simulink library "inp"  (R2021b)
settings: Solver=VariableStepAuto  StartTime=0.0  StopTime=10.0  RelTol=1e-3
undefined symbols (not defined in the file): C_TASK_5MS_S, FALSE, KINP_AcoreReadyToSlp_flg_ovrdflg, KINP_AcoreReadyToSlp_flg_ovrdval, KINP_AllowMovThd_OTA_enum_ovrdflg, KINP_AllowMovThd_OTA_enum_ovrdval, KINP_APSAngleTarget_Deg_ovrdflg, KINP_APSAngleTarget_Deg_ovrdval, KINP_APSDecReq_mps2_ovrdflg, KINP_APSDecReq_mps2_ovrdval, KINP_APSDecReqA_flg_ovrdflg, KINP_APSDecReqA_flg_ovrdval, KINP_APSDFLL_cm_ovrdflg, KINP_APSDFLL_cm_ovrdval, KINP_APSDFLR_cm_ovrdflg, KINP_APSDFLR_cm_ovrdval, KINP_APSDRLL_cm_ovrdflg, KINP_APSDRLL_cm_ovrdval, KINP_APSDRLR_cm_ovrdflg, KINP_APSDRLR_cm_ovrdval, KINP_APSExitCondition_enum_ovrdflg, KINP_APSExitCondition_enum_ovrdval, KINP_APSHWVer_enum_ovrdflg, KINP_APSHWVer_enum_ovrdval, KINP_APSProgressPCT_pct_ovrdflg, KINP_APSProgressPCT_pct_ovrdval, KINP_APSReq_enum_ovrdflg, KINP_APSReq_enum_ovrdval, KINP_APSRQDisplay_enum_ovrdflg, KINP_APSRQDisplay_enum_ovrdval, KINP_APSRqEPASCtrl_flg_ovrdflg, KINP_APSRqEPASCtrl_flg_ovrdval, KINP_APSShiftPosnReq_enum_ovrdval, KINP_APSShiftPosnReq_enum_ovrflg, KINP_APSSpeedCMD_kph_ovrdval, KINP_APSSpeedCMD_kph_ovrflg, KINP_APSStaSystem_enum_ovrdflg, KINP_APSStaSystem_enum_ovrdval, KINP_APSSWVer_enum_ovrdflg, KINP_APSSWVer_enum_ovrdval, KINP_APSVMCReqA_flg_ovrdval, KINP_APSVMCReqA_flg_ovrflg, KINP_APSVRqEPASCtrl_flg_ovrdflg, KINP_APSVRqEPASCtrl_flg_ovrdval, KINP_AuxBattVolmV_mV_ovrdflg, KINP_AuxBattVolmV_mV_ovrdval, KINP_CAASSta_enum_ovrdflg, KINP_CAASSta_enum_ovrdval, KINP_CAASVMCReqA_flg_ovrdval, KINP_CAASVMCReqA_flg_ovrflg, KINP_Chime_enum_ovrdflg, KINP_Chime_enum_ovrdval, KINP_ClearDTCcmd_flg_ovrdflg, KINP_ClearDTCcmd_flg_ovrdval, KINP_EvccAplusPwrUpReq_flg_ovrdflg, KINP_EvccAplusPwrUpReq_flg_ovrdval, KINP_LFID_raw_ovrdval, KINP_LFID_raw_ovrflg, KINP_LRID_raw_ovrdval, KINP_MemOffsetAccX_raw16_ovrdflg ... (+118)
libraries: FVT_lib x503, hcu_lib x1
(part 11 of 16)

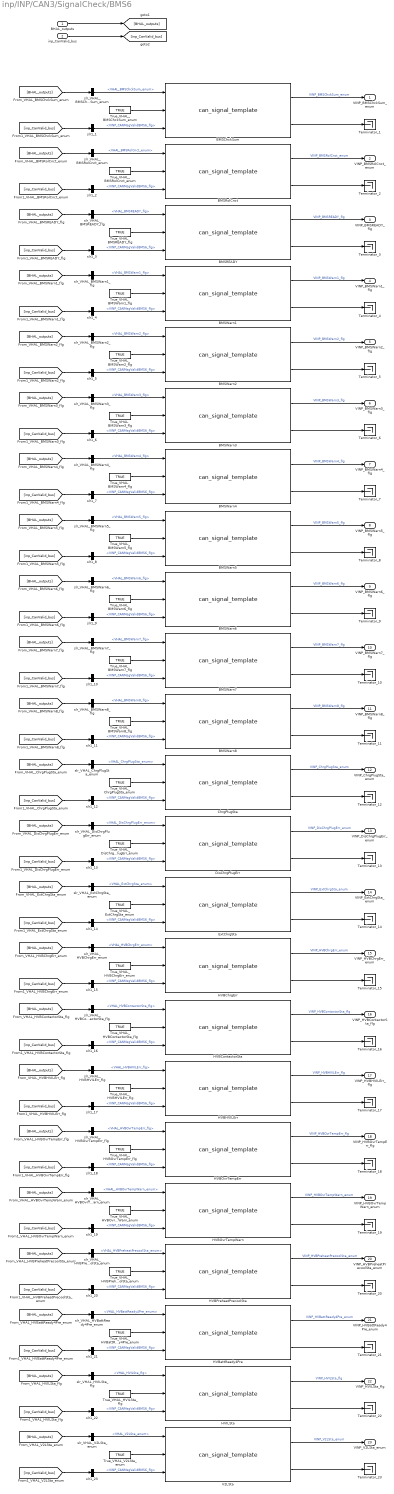
== system inp/INP/CAN3/SignalCheck/BMS6 ==
  BHAL_outputs : Inport
  inp_CanValid_bus : Inport  Port=2
  BMSChckSum : FVT_lib/inp/can_signal_template  SystemSampleTime=-1  VariantActivationTime=update diagram  Latency=0  AutoFrameSizeCalculation=off
      link override defval: Value=KINP_BMSChckSum_enum_defval
      link override ovrdflg: Value=KINP_BMSChckSum_enum_ovrdflg
      link override ovrdval: Value=KINP_BMSChckSum_enum_ovrdval
  BMSREADY : FVT_lib/inp/can_signal_template  SystemSampleTime=-1  VariantActivationTime=update diagram  Latency=0  AutoFrameSizeCalculation=off
      link override defval: Value=KINP_BMSREADY_flg_defval
      link override ovrdflg: Value=KINP_BMSREADY_flg_ovrdflg
      link override ovrdval: Value=KINP_BMSREADY_flg_ovrdval
  BMSRolCnct : FVT_lib/inp/can_signal_template  SystemSampleTime=-1  VariantActivationTime=update diagram  Latency=0  AutoFrameSizeCalculation=off
      link override defval: Value=KINP_BMSRolCnct_enum_defval
      link override ovrdflg: Value=KINP_BMSRolCnct_enum_ovrdflg
      link override ovrdval: Value=KINP_BMSRolCnct_enum_ovrdval
  BMSWarn1 : FVT_lib/inp/can_signal_template  SystemSampleTime=-1  VariantActivationTime=update diagram  Latency=0  AutoFrameSizeCalculation=off
      link override defval: Value=KINP_BMSWarn1_flg_defval
      link override ovrdflg: Value=KINP_BMSWarn1_flg_ovrdflg
      link override ovrdval: Value=KINP_BMSWarn1_flg_ovrdval
  BMSWarn2 : FVT_lib/inp/can_signal_template  SystemSampleTime=-1  VariantActivationTime=update diagram  Latency=0  AutoFrameSizeCalculation=off
      link override defval: Value=KINP_BMSWarn2_flg_defval
      link override ovrdflg: Value=KINP_BMSWarn2_flg_ovrdflg
      link override ovrdval: Value=KINP_BMSWarn2_flg_ovrdval
  BMSWarn3 : FVT_lib/inp/can_signal_template  SystemSampleTime=-1  VariantActivationTime=update diagram  Latency=0  AutoFrameSizeCalculation=off
      link override defval: Value=KINP_BMSWarn3_flg_defval
      link override ovrdflg: Value=KINP_BMSWarn3_flg_ovrdflg
      link override ovrdval: Value=KINP_BMSWarn3_flg_ovrdval
  BMSWarn4 : FVT_lib/inp/can_signal_template  SystemSampleTime=-1  VariantActivationTime=update diagram  Latency=0  AutoFrameSizeCalculation=off
      link override defval: Value=KINP_BMSWarn4_flg_defval
      link override ovrdflg: Value=KINP_BMSWarn4_flg_ovrdflg
      link override ovrdval: Value=KINP_BMSWarn4_flg_ovrdval
  BMSWarn5 : FVT_lib/inp/can_signal_template  SystemSampleTime=-1  VariantActivationTime=update diagram  Latency=0  AutoFrameSizeCalculation=off
      link override defval: Value=KINP_BMSWarn5_flg_defval
      link override ovrdflg: Value=KINP_BMSWarn5_flg_ovrdflg
      link override ovrdval: Value=KINP_BMSWarn5_flg_ovrdval
  BMSWarn6 : FVT_lib/inp/can_signal_template  SystemSampleTime=-1  VariantActivationTime=update diagram  Latency=0  AutoFrameSizeCalculation=off
      link override defval: Value=KINP_BMSWarn6_flg_defval
      link override ovrdflg: Value=KINP_BMSWarn6_flg_ovrdflg
      link override ovrdval: Value=KINP_BMSWarn6_flg_ovrdval
  BMSWarn7 : FVT_lib/inp/can_signal_template  SystemSampleTime=-1  VariantActivationTime=update diagram  Latency=0  AutoFrameSizeCalculation=off
      link override defval: Value=KINP_BMSWarn7_flg_defval
      link override ovrdflg: Value=KINP_BMSWarn7_flg_ovrdflg
      link override ovrdval: Value=KINP_BMSWarn7_flg_ovrdval
  BMSWarn8 : FVT_lib/inp/can_signal_template  SystemSampleTime=-1  VariantActivationTime=update diagram  Latency=0  AutoFrameSizeCalculation=off
      link override defval: Value=KINP_BMSWarn8_flg_defval
      link override ovrdflg: Value=KINP_BMSWarn8_flg_ovrdflg
      link override ovrdval: Value=KINP_BMSWarn8_flg_ovrdval
  ChrgPlugSta : FVT_lib/inp/can_signal_template  SystemSampleTime=-1  VariantActivationTime=update diagram  Latency=0  AutoFrameSizeCalculation=off
      link override defval: Value=KINP_ChrgPlugSta_enum_defval
      link override ovrdflg: Value=KINP_ChrgPlugSta_enum_ovrdflg
      link override ovrdval: Value=KINP_ChrgPlugSta_enum_ovrdval
  DisChrgPlugErr : FVT_lib/inp/can_signal_template  SystemSampleTime=-1  VariantActivationTime=update diagram  Latency=0  AutoFrameSizeCalculation=off
      link override defval: Value=KINP_DisChrgPlugErr_enum_defval
      link override ovrdflg: Value=KINP_DisChrgPlugErr_enum_ovrdflg
      link override ovrdval: Value=KINP_DisChrgPlugErr_enum_ovrdval
  ExtChrgSta : FVT_lib/inp/can_signal_template  SystemSampleTime=-1  VariantActivationTime=update diagram  Latency=0  AutoFrameSizeCalculation=off
      link override defval: Value=KINP_ExtChrgSta_enum_defval
      link override ovrdflg: Value=KINP_ExtChrgSta_enum_ovrdflg
      link override ovrdval: Value=KINP_ExtChrgSta_enum_ovrdval
  HVBChrgErr : FVT_lib/inp/can_signal_template  SystemSampleTime=-1  VariantActivationTime=update diagram  Latency=0  AutoFrameSizeCalculation=off
      link override defval: Value=KINP_HVBChrgErr_enum_defval
      link override ovrdflg: Value=KINP_HVBChrgErr_enum_ovrdflg
      link override ovrdval: Value=KINP_HVBChrgErr_enum_ovrdval
  HVBContactorSta : FVT_lib/inp/can_signal_template  SystemSampleTime=-1  VariantActivationTime=update diagram  Latency=0  AutoFrameSizeCalculation=off
      link override defval: Value=KINP_HVBContactorSta_flg_defval
      link override ovrdflg: Value=KINP_HVBContactorSta_flg_ovrdflg
      link override ovrdval: Value=KINP_HVBContactorSta_flg_ovrdval
  HVBHVILErr : FVT_lib/inp/can_signal_template  SystemSampleTime=-1  VariantActivationTime=update diagram  Latency=0  AutoFrameSizeCalculation=off
      link override defval: Value=KINP_HVBHVILErr_flg_defval
      link override ovrdflg: Value=KINP_HVBHVILErr_flg_ovrdflg
      link override ovrdval: Value=KINP_HVBHVILErr_flg_ovrdval
  HVBOvrTempErr : FVT_lib/inp/can_signal_template  SystemSampleTime=-1  VariantActivationTime=update diagram  Latency=0  AutoFrameSizeCalculation=off
      link override defval: Value=KINP_HVBOvrTempErr_flg_defval
      link override ovrdflg: Value=KINP_HVBOvrTempErr_flg_ovrdflg
      link override ovrdval: Value=KINP_HVBOvrTempErr_flg_ovrdval
  HVBOvrTempWarn : FVT_lib/inp/can_signal_template  SystemSampleTime=-1  VariantActivationTime=update diagram  Latency=0  AutoFrameSizeCalculation=off
      link override defval: Value=KINP_HVBOvrTempWarn_enum_defval
      link override ovrdflg: Value=KINP_HVBOvrTempWarn_enum_ovrdflg
      link override ovrdval: Value=KINP_HVBOvrTempWarn_enum_ovrdval
  HVBPreheatPrecoolSta : FVT_lib/inp/can_signal_template  SystemSampleTime=-1  VariantActivationTime=update diagram  Latency=0  AutoFrameSizeCalculation=off
      link override defval: Value=KINP_HVBPreheatPrecoolSta_enum_defval
      link override ovrdflg: Value=KINP_HVBPreheatPrecoolSta_enum_ovrdflg
      link override ovrdval: Value=KINP_HVBPreheatPrecoolSta_enum_ovrdval
  HVBattReady4Pre : FVT_lib/inp/can_signal_template  SystemSampleTime=-1  VariantActivationTime=update diagram  Latency=0  AutoFrameSizeCalculation=off
      link override defval: Value=KINP_HVBattReady4Pre_enum_defval
      link override ovrdflg: Value=KINP_HVBattReady4Pre_enum_ovrdflg
      link override ovrdval: Value=KINP_HVBattReady4Pre_enum_ovrdval
  HVILSta : FVT_lib/inp/can_signal_template  SystemSampleTime=-1  VariantActivationTime=update diagram  Latency=0  AutoFrameSizeCalculation=off
      link override defval: Value=KINP_HVILSta_flg_defval
      link override ovrdflg: Value=KINP_HVILSta_flg_ovrdflg
      link override ovrdval: Value=KINP_HVILSta_flg_ovrdval
  Terminator_{1..23} (23 alike) : Terminator
  True_VHAL_BMSChckSum_enum : Constant  Value=TRUE  OutDataTypeStr=boolean
  True_VHAL_BMSREADY_flg : Constant  Value=TRUE  OutDataTypeStr=boolean
  True_VHAL_BMSRolCnct_enum : Constant  Value=TRUE  OutDataTypeStr=boolean
  True_VHAL_BMSWarn1_flg : Constant  Value=TRUE  OutDataTypeStr=boolean
  True_VHAL_BMSWarn2_flg : Constant  Value=TRUE  OutDataTypeStr=boolean
  True_VHAL_BMSWarn3_flg : Constant  Value=TRUE  OutDataTypeStr=boolean
  True_VHAL_BMSWarn4_flg : Constant  Value=TRUE  OutDataTypeStr=boolean
  True_VHAL_BMSWarn5_flg : Constant  Value=TRUE  OutDataTypeStr=boolean
  True_VHAL_BMSWarn6_flg : Constant  Value=TRUE  OutDataTypeStr=boolean
  True_VHAL_BMSWarn7_flg : Constant  Value=TRUE  OutDataTypeStr=boolean
  True_VHAL_BMSWarn8_flg : Constant  Value=TRUE  OutDataTypeStr=boolean
  True_VHAL_ChrgPlugSta_enum : Constant  Value=TRUE  OutDataTypeStr=boolean
  True_VHAL_DisChrgPlugErr_enum : Constant  Value=TRUE  OutDataTypeStr=boolean
  True_VHAL_ExtChrgSta_enum : Constant  Value=TRUE  OutDataTypeStr=boolean
  True_VHAL_HVBChrgErr_enum : Constant  Value=TRUE  OutDataTypeStr=boolean
  True_VHAL_HVBContactorSta_flg : Constant  Value=TRUE  OutDataTypeStr=boolean
  True_VHAL_HVBHVILErr_flg : Constant  Value=TRUE  OutDataTypeStr=boolean
  True_VHAL_HVBOvrTempErr_flg : Constant  Value=TRUE  OutDataTypeStr=boolean
  True_VHAL_HVBOvrTempWarn_enum : Constant  Value=TRUE  OutDataTypeStr=boolean
  True_VHAL_HVBPreheatPrecoolSta_enum : Constant  Value=TRUE  OutDataTypeStr=boolean
  True_VHAL_HVBattReady4Pre_enum : Constant  Value=TRUE  OutDataTypeStr=boolean
  True_VHAL_HVILSta_flg : Constant  Value=TRUE  OutDataTypeStr=boolean
  True_VHAL_V2LSta_enum : Constant  Value=TRUE  OutDataTypeStr=boolean
  V2LSta : FVT_lib/inp/can_signal_template  SystemSampleTime=-1  VariantActivationTime=update diagram  Latency=0  AutoFrameSizeCalculation=off
      link override defval: Value=KINP_V2LSta_enum_defval
      link override ovrdflg: Value=KINP_V2LSta_enum_ovrdflg
      link override ovrdval: Value=KINP_V2LSta_enum_ovrdval
  slr1_{1..23} (23 alike) : BusSelector  OutputSignals=VINP_CANMsgValidBMS6_flg
  slr_VHAL_BMSChckSum_enum : BusSelector  OutputSignals=VHAL_BMSChckSum_enum
  slr_VHAL_BMSREADY_flg : BusSelector  OutputSignals=VHAL_BMSREADY_flg
  slr_VHAL_BMSRolCnct_enum : BusSelector  OutputSignals=VHAL_BMSRolCnct_enum
  slr_VHAL_BMSWarn1_flg : BusSelector  OutputSignals=VHAL_BMSWarn1_flg
  slr_VHAL_BMSWarn2_flg : BusSelector  OutputSignals=VHAL_BMSWarn2_flg
  slr_VHAL_BMSWarn3_flg : BusSelector  OutputSignals=VHAL_BMSWarn3_flg
  slr_VHAL_BMSWarn4_flg : BusSelector  OutputSignals=VHAL_BMSWarn4_flg
  slr_VHAL_BMSWarn5_flg : BusSelector  OutputSignals=VHAL_BMSWarn5_flg
  slr_VHAL_BMSWarn6_flg : BusSelector  OutputSignals=VHAL_BMSWarn6_flg
  slr_VHAL_BMSWarn7_flg : BusSelector  OutputSignals=VHAL_BMSWarn7_flg
  slr_VHAL_BMSWarn8_flg : BusSelector  OutputSignals=VHAL_BMSWarn8_flg
  slr_VHAL_ChrgPlugSta_enum : BusSelector  OutputSignals=VHAL_ChrgPlugSta_enum
  slr_VHAL_DisChrgPlugErr_enum : BusSelector  OutputSignals=VHAL_DisChrgPlugErr_enum
  slr_VHAL_ExtChrgSta_enum : BusSelector  OutputSignals=VHAL_ExtChrgSta_enum
  slr_VHAL_HVBChrgErr_enum : BusSelector  OutputSignals=VHAL_HVBChrgErr_enum
  slr_VHAL_HVBContactorSta_flg : BusSelector  OutputSignals=VHAL_HVBContactorSta_flg
  slr_VHAL_HVBHVILErr_flg : BusSelector  OutputSignals=VHAL_HVBHVILErr_flg
  slr_VHAL_HVBOvrTempErr_flg : BusSelector  OutputSignals=VHAL_HVBOvrTempErr_flg
  slr_VHAL_HVBOvrTempWarn_enum : BusSelector  OutputSignals=VHAL_HVBOvrTempWarn_enum
  slr_VHAL_HVBPreheatPrecoolSta_enum : BusSelector  OutputSignals=VHAL_HVBPreheatPrecoolSta_enum
  slr_VHAL_HVBattReady4Pre_enum : BusSelector  OutputSignals=VHAL_HVBattReady4Pre_enum
  slr_VHAL_HVILSta_flg : BusSelector  OutputSignals=VHAL_HVILSta_flg
  slr_VHAL_V2LSta_enum : BusSelector  OutputSignals=VHAL_V2LSta_enum
  VINP_BMSChckSum_enum : Outport
  VINP_BMSRolCnct_enum : Outport  Port=2
  VINP_BMSREADY_flg : Outport  Port=3
  VINP_BMSWarn1_flg : Outport  Port=4
  VINP_BMSWarn2_flg : Outport  Port=5
  VINP_BMSWarn3_flg : Outport  Port=6
  VINP_BMSWarn4_flg : Outport  Port=7
  VINP_BMSWarn5_flg : Outport  Port=8
  VINP_BMSWarn6_flg : Outport  Port=9
  VINP_BMSWarn7_flg : Outport  Port=10
  VINP_BMSWarn8_flg : Outport  Port=11
  VINP_ChrgPlugSta_enum : Outport  Port=12
  VINP_DisChrgPlugErr_enum : Outport  Port=13
  VINP_ExtChrgSta_enum : Outport  Port=14
  VINP_HVBChrgErr_enum : Outport  Port=15
  VINP_HVBContactorSta_flg : Outport  Port=16
  VINP_HVBHVILErr_flg : Outport  Port=17
  VINP_HVBOvrTempErr_flg : Outport  Port=18
  VINP_HVBOvrTempWarn_enum : Outport  Port=19
  VINP_HVBPreheatPrecoolSta_enum : Outport  Port=20
  VINP_HVBattReady4Pre_enum : Outport  Port=21
  VINP_HVILSta_flg : Outport  Port=22
  VINP_V2LSta_enum : Outport  Port=23
  wires:
  BHAL_outputs/1 -> [BHAL_outputs]
  inp_CanValid_bus/1 -> [inp_CanValid_bus]
  [BHAL_outputs] -> slr_VHAL_BMSChckSum_enum/1
  slr_VHAL_BMSChckSum_enum/1 -> BMSChckSum/1  "<VHAL_BMSChckSum_enum>"
  True_VHAL_BMSChckSum_enum/1 -> BMSChckSum/2
  [inp_CanValid_bus] -> slr1_1/1
  slr1_1/1 -> BMSChckSum/3  "<VINP_CANMsgValidBMS6_flg>"
  BMSChckSum/1 -> VINP_BMSChckSum_enum/1  "VINP_BMSChckSum_enum"
  BMSChckSum/2 -> Terminator_1/1
  [BHAL_outputs] -> slr_VHAL_BMSRolCnct_enum/1
  slr_VHAL_BMSRolCnct_enum/1 -> BMSRolCnct/1  "<VHAL_BMSRolCnct_enum>"
  True_VHAL_BMSRolCnct_enum/1 -> BMSRolCnct/2
  [inp_CanValid_bus] -> slr1_2/1
  slr1_2/1 -> BMSRolCnct/3  "<VINP_CANMsgValidBMS6_flg>"
  BMSRolCnct/1 -> VINP_BMSRolCnct_enum/1  "VINP_BMSRolCnct_enum"
  BMSRolCnct/2 -> Terminator_2/1
  [BHAL_outputs] -> slr_VHAL_BMSREADY_flg/1
  slr_VHAL_BMSREADY_flg/1 -> BMSREADY/1  "<VHAL_BMSREADY_flg>"
  True_VHAL_BMSREADY_flg/1 -> BMSREADY/2
  [inp_CanValid_bus] -> slr1_3/1
  slr1_3/1 -> BMSREADY/3  "<VINP_CANMsgValidBMS6_flg>"
  BMSREADY/1 -> VINP_BMSREADY_flg/1  "VINP_BMSREADY_flg"
  BMSREADY/2 -> Terminator_3/1
  [BHAL_outputs] -> slr_VHAL_BMSWarn1_flg/1
  slr_VHAL_BMSWarn1_flg/1 -> BMSWarn1/1  "<VHAL_BMSWarn1_flg>"
  True_VHAL_BMSWarn1_flg/1 -> BMSWarn1/2
  [inp_CanValid_bus] -> slr1_4/1
  slr1_4/1 -> BMSWarn1/3  "<VINP_CANMsgValidBMS6_flg>"
  BMSWarn1/1 -> VINP_BMSWarn1_flg/1  "VINP_BMSWarn1_flg"
  BMSWarn1/2 -> Terminator_4/1
  [BHAL_outputs] -> slr_VHAL_BMSWarn2_flg/1
  slr_VHAL_BMSWarn2_flg/1 -> BMSWarn2/1  "<VHAL_BMSWarn2_flg>"
  True_VHAL_BMSWarn2_flg/1 -> BMSWarn2/2
  [inp_CanValid_bus] -> slr1_5/1
  slr1_5/1 -> BMSWarn2/3  "<VINP_CANMsgValidBMS6_flg>"
  BMSWarn2/1 -> VINP_BMSWarn2_flg/1  "VINP_BMSWarn2_flg"
  BMSWarn2/2 -> Terminator_5/1
  [BHAL_outputs] -> slr_VHAL_BMSWarn3_flg/1
  slr_VHAL_BMSWarn3_flg/1 -> BMSWarn3/1  "<VHAL_BMSWarn3_flg>"
  True_VHAL_BMSWarn3_flg/1 -> BMSWarn3/2
  [inp_CanValid_bus] -> slr1_6/1
  slr1_6/1 -> BMSWarn3/3  "<VINP_CANMsgValidBMS6_flg>"
  BMSWarn3/1 -> VINP_BMSWarn3_flg/1  "VINP_BMSWarn3_flg"
  BMSWarn3/2 -> Terminator_6/1
  [BHAL_outputs] -> slr_VHAL_BMSWarn4_flg/1
  slr_VHAL_BMSWarn4_flg/1 -> BMSWarn4/1  "<VHAL_BMSWarn4_flg>"
  True_VHAL_BMSWarn4_flg/1 -> BMSWarn4/2
  [inp_CanValid_bus] -> slr1_7/1
  slr1_7/1 -> BMSWarn4/3  "<VINP_CANMsgValidBMS6_flg>"
  BMSWarn4/1 -> VINP_BMSWarn4_flg/1  "VINP_BMSWarn4_flg"
  BMSWarn4/2 -> Terminator_7/1
  [BHAL_outputs] -> slr_VHAL_BMSWarn5_flg/1
  slr_VHAL_BMSWarn5_flg/1 -> BMSWarn5/1  "<VHAL_BMSWarn5_flg>"
  True_VHAL_BMSWarn5_flg/1 -> BMSWarn5/2
  [inp_CanValid_bus] -> slr1_8/1
  slr1_8/1 -> BMSWarn5/3  "<VINP_CANMsgValidBMS6_flg>"
  BMSWarn5/1 -> VINP_BMSWarn5_flg/1  "VINP_BMSWarn5_flg"
  BMSWarn5/2 -> Terminator_8/1
  [BHAL_outputs] -> slr_VHAL_BMSWarn6_flg/1
  slr_VHAL_BMSWarn6_flg/1 -> BMSWarn6/1  "<VHAL_BMSWarn6_flg>"
  True_VHAL_BMSWarn6_flg/1 -> BMSWarn6/2
  [inp_CanValid_bus] -> slr1_9/1
  slr1_9/1 -> BMSWarn6/3  "<VINP_CANMsgValidBMS6_flg>"
  BMSWarn6/1 -> VINP_BMSWarn6_flg/1  "VINP_BMSWarn6_flg"
  BMSWarn6/2 -> Terminator_9/1
  [BHAL_outputs] -> slr_VHAL_BMSWarn7_flg/1
  slr_VHAL_BMSWarn7_flg/1 -> BMSWarn7/1  "<VHAL_BMSWarn7_flg>"
  True_VHAL_BMSWarn7_flg/1 -> BMSWarn7/2
  [inp_CanValid_bus] -> slr1_10/1
  slr1_10/1 -> BMSWarn7/3  "<VINP_CANMsgValidBMS6_flg>"
  BMSWarn7/1 -> VINP_BMSWarn7_flg/1  "VINP_BMSWarn7_flg"
  BMSWarn7/2 -> Terminator_10/1
  [BHAL_outputs] -> slr_VHAL_BMSWarn8_flg/1
  slr_VHAL_BMSWarn8_flg/1 -> BMSWarn8/1  "<VHAL_BMSWarn8_flg>"
  True_VHAL_BMSWarn8_flg/1 -> BMSWarn8/2
  [inp_CanValid_bus] -> slr1_11/1
  slr1_11/1 -> BMSWarn8/3  "<VINP_CANMsgValidBMS6_flg>"
  BMSWarn8/1 -> VINP_BMSWarn8_flg/1  "VINP_BMSWarn8_flg"
  BMSWarn8/2 -> Terminator_11/1
  [BHAL_outputs] -> slr_VHAL_ChrgPlugSta_enum/1
  slr_VHAL_ChrgPlugSta_enum/1 -> ChrgPlugSta/1  "<VHAL_ChrgPlugSta_enum>"
  True_VHAL_ChrgPlugSta_enum/1 -> ChrgPlugSta/2
  [inp_CanValid_bus] -> slr1_12/1
  slr1_12/1 -> ChrgPlugSta/3  "<VINP_CANMsgValidBMS6_flg>"
  ChrgPlugSta/1 -> VINP_ChrgPlugSta_enum/1  "VINP_ChrgPlugSta_enum"
  ChrgPlugSta/2 -> Terminator_12/1
  [BHAL_outputs] -> slr_VHAL_DisChrgPlugErr_enum/1
  slr_VHAL_DisChrgPlugErr_enum/1 -> DisChrgPlugErr/1  "<VHAL_DisChrgPlugErr_enum>"
  True_VHAL_DisChrgPlugErr_enum/1 -> DisChrgPlugErr/2
  [inp_CanValid_bus] -> slr1_13/1
  slr1_13/1 -> DisChrgPlugErr/3  "<VINP_CANMsgValidBMS6_flg>"
  DisChrgPlugErr/1 -> VINP_DisChrgPlugErr_enum/1  "VINP_DisChrgPlugErr_enum"
  DisChrgPlugErr/2 -> Terminator_13/1
  [BHAL_outputs] -> slr_VHAL_ExtChrgSta_enum/1
  slr_VHAL_ExtChrgSta_enum/1 -> ExtChrgSta/1  "<VHAL_ExtChrgSta_enum>"
  True_VHAL_ExtChrgSta_enum/1 -> ExtChrgSta/2
  [inp_CanValid_bus] -> slr1_14/1
  slr1_14/1 -> ExtChrgSta/3  "<VINP_CANMsgValidBMS6_flg>"
  ExtChrgSta/1 -> VINP_ExtChrgSta_enum/1  "VINP_ExtChrgSta_enum"
  ExtChrgSta/2 -> Terminator_14/1
  [BHAL_outputs] -> slr_VHAL_HVBChrgErr_enum/1
  slr_VHAL_HVBChrgErr_enum/1 -> HVBChrgErr/1  "<VHAL_HVBChrgErr_enum>"
  True_VHAL_HVBChrgErr_enum/1 -> HVBChrgErr/2
  [inp_CanValid_bus] -> slr1_15/1
  slr1_15/1 -> HVBChrgErr/3  "<VINP_CANMsgValidBMS6_flg>"
  HVBChrgErr/1 -> VINP_HVBChrgErr_enum/1  "VINP_HVBChrgErr_enum"
  HVBChrgErr/2 -> Terminator_15/1
  [BHAL_outputs] -> slr_VHAL_HVBContactorSta_flg/1
  slr_VHAL_HVBContactorSta_flg/1 -> HVBContactorSta/1  "<VHAL_HVBContactorSta_flg>"
  True_VHAL_HVBContactorSta_flg/1 -> HVBContactorSta/2
  [inp_CanValid_bus] -> slr1_16/1
  slr1_16/1 -> HVBContactorSta/3  "<VINP_CANMsgValidBMS6_flg>"
  HVBContactorSta/1 -> VINP_HVBContactorSta_flg/1  "VINP_HVBContactorSta_flg"
  HVBContactorSta/2 -> Terminator_16/1
  [BHAL_outputs] -> slr_VHAL_HVBHVILErr_flg/1
  slr_VHAL_HVBHVILErr_flg/1 -> HVBHVILErr/1  "<VHAL_HVBHVILErr_flg>"
  True_VHAL_HVBHVILErr_flg/1 -> HVBHVILErr/2
  [inp_CanValid_bus] -> slr1_17/1
  slr1_17/1 -> HVBHVILErr/3  "<VINP_CANMsgValidBMS6_flg>"
  HVBHVILErr/1 -> VINP_HVBHVILErr_flg/1  "VINP_HVBHVILErr_flg"
  HVBHVILErr/2 -> Terminator_17/1
  [BHAL_outputs] -> slr_VHAL_HVBOvrTempErr_flg/1
  slr_VHAL_HVBOvrTempErr_flg/1 -> HVBOvrTempErr/1  "<VHAL_HVBOvrTempErr_flg>"
  True_VHAL_HVBOvrTempErr_flg/1 -> HVBOvrTempErr/2
  [inp_CanValid_bus] -> slr1_18/1
  slr1_18/1 -> HVBOvrTempErr/3  "<VINP_CANMsgValidBMS6_flg>"
  HVBOvrTempErr/1 -> VINP_HVBOvrTempErr_flg/1  "VINP_HVBOvrTempErr_flg"
  HVBOvrTempErr/2 -> Terminator_18/1
  [BHAL_outputs] -> slr_VHAL_HVBOvrTempWarn_enum/1
  slr_VHAL_HVBOvrTempWarn_enum/1 -> HVBOvrTempWarn/1  "<VHAL_HVBOvrTempWarn_enum>"
  True_VHAL_HVBOvrTempWarn_enum/1 -> HVBOvrTempWarn/2
  [inp_CanValid_bus] -> slr1_19/1
  slr1_19/1 -> HVBOvrTempWarn/3  "<VINP_CANMsgValidBMS6_flg>"
  HVBOvrTempWarn/1 -> VINP_HVBOvrTempWarn_enum/1  "VINP_HVBOvrTempWarn_enum"
  HVBOvrTempWarn/2 -> Terminator_19/1
  [BHAL_outputs] -> slr_VHAL_HVBPreheatPrecoolSta_enum/1
  slr_VHAL_HVBPreheatPrecoolSta_enum/1 -> HVBPreheatPrecoolSta/1  "<VHAL_HVBPreheatPrecoolSta_enum>"
  True_VHAL_HVBPreheatPrecoolSta_enum/1 -> HVBPreheatPrecoolSta/2
  [inp_CanValid_bus] -> slr1_20/1
  slr1_20/1 -> HVBPreheatPrecoolSta/3  "<VINP_CANMsgValidBMS6_flg>"
  HVBPreheatPrecoolSta/1 -> VINP_HVBPreheatPrecoolSta_enum/1  "VINP_HVBPreheatPrecoolSta_enum"
  HVBPreheatPrecoolSta/2 -> Terminator_20/1
  [BHAL_outputs] -> slr_VHAL_HVBattReady4Pre_enum/1
  slr_VHAL_HVBattReady4Pre_enum/1 -> HVBattReady4Pre/1  "<VHAL_HVBattReady4Pre_enum>"
  True_VHAL_HVBattReady4Pre_enum/1 -> HVBattReady4Pre/2
  [inp_CanValid_bus] -> slr1_21/1
  slr1_21/1 -> HVBattReady4Pre/3  "<VINP_CANMsgValidBMS6_flg>"
  HVBattReady4Pre/1 -> VINP_HVBattReady4Pre_enum/1  "VINP_HVBattReady4Pre_enum"
  HVBattReady4Pre/2 -> Terminator_21/1
  [BHAL_outputs] -> slr_VHAL_HVILSta_flg/1
  slr_VHAL_HVILSta_flg/1 -> HVILSta/1  "<VHAL_HVILSta_flg>"
  True_VHAL_HVILSta_flg/1 -> HVILSta/2
  [inp_CanValid_bus] -> slr1_22/1
  slr1_22/1 -> HVILSta/3  "<VINP_CANMsgValidBMS6_flg>"
  HVILSta/1 -> VINP_HVILSta_flg/1  "VINP_HVILSta_flg"
  HVILSta/2 -> Terminator_22/1
  [BHAL_outputs] -> slr_VHAL_V2LSta_enum/1
  slr_VHAL_V2LSta_enum/1 -> V2LSta/1  "<VHAL_V2LSta_enum>"
  True_VHAL_V2LSta_enum/1 -> V2LSta/2
  [inp_CanValid_bus] -> slr1_23/1
  slr1_23/1 -> V2LSta/3  "<VINP_CANMsgValidBMS6_flg>"
  V2LSta/1 -> VINP_V2LSta_enum/1  "VINP_V2LSta_enum"
  V2LSta/2 -> Terminator_23/1

== system inp/INP/CAN3/SignalCheck/BMS8 ==
  BHAL_outputs : Inport
  inp_CanValid_bus : Inport  Port=2
  MainRlyNegSta : FVT_lib/inp/can_signal_template  SystemSampleTime=-1  VariantActivationTime=update diagram  Latency=0  AutoFrameSizeCalculation=off
      link override defval: Value=KINP_MainRlyNegSta_enum_defval
      link override ovrdflg: Value=KINP_MainRlyNegSta_enum_ovrdflg
      link override ovrdval: Value=KINP_MainRlyNegSta_enum_ovrdval
  MainRlyPosSta : FVT_lib/inp/can_signal_template  SystemSampleTime=-1  VariantActivationTime=update diagram  Latency=0  AutoFrameSizeCalculation=off
      link override defval: Value=KINP_MainRlyPosSta_enum_defval
      link override ovrdflg: Value=KINP_MainRlyPosSta_enum_ovrdflg
      link override ovrdval: Value=KINP_MainRlyPosSta_enum_ovrdval
  Terminator_1 : Terminator
  Terminator_2 : Terminator
  True_VHAL_MainRlyNegSta_enum : Constant  Value=TRUE  OutDataTypeStr=boolean
  True_VHAL_MainRlyPosSta_enum : Constant  Value=TRUE  OutDataTypeStr=boolean
  slr1_1 : BusSelector  OutputSignals=VINP_CANMsgValidBMS8_flg
  slr1_2 : BusSelector  OutputSignals=VINP_CANMsgValidBMS8_flg
  slr_VHAL_MainRlyNegSta_enum : BusSelector  OutputSignals=VHAL_MainRlyNegSta_enum
  slr_VHAL_MainRlyPosSta_enum : BusSelector  OutputSignals=VHAL_MainRlyPosSta_enum
  VINP_MainRlyNegSta_enum : Outport
  VINP_MainRlyPosSta_enum : Outport  Port=2
  wires:
  BHAL_outputs/1 -> [BHAL_outputs]
  inp_CanValid_bus/1 -> [inp_CanValid_bus]
  [BHAL_outputs] -> slr_VHAL_MainRlyNegSta_enum/1
  slr_VHAL_MainRlyNegSta_enum/1 -> MainRlyNegSta/1  "<VHAL_MainRlyNegSta_enum>"
  True_VHAL_MainRlyNegSta_enum/1 -> MainRlyNegSta/2
  [inp_CanValid_bus] -> slr1_1/1
  slr1_1/1 -> MainRlyNegSta/3  "<VINP_CANMsgValidBMS8_flg>"
  MainRlyNegSta/1 -> VINP_MainRlyNegSta_enum/1  "VINP_MainRlyNegSta_enum"
  MainRlyNegSta/2 -> Terminator_1/1
  [BHAL_outputs] -> slr_VHAL_MainRlyPosSta_enum/1
  slr_VHAL_MainRlyPosSta_enum/1 -> MainRlyPosSta/1  "<VHAL_MainRlyPosSta_enum>"
  True_VHAL_MainRlyPosSta_enum/1 -> MainRlyPosSta/2
  [inp_CanValid_bus] -> slr1_2/1
  slr1_2/1 -> MainRlyPosSta/3  "<VINP_CANMsgValidBMS8_flg>"
  MainRlyPosSta/1 -> VINP_MainRlyPosSta_enum/1  "VINP_MainRlyPosSta_enum"
  MainRlyPosSta/2 -> Terminator_2/1

== system inp/INP/CAN3/SignalCheck/CCU1 ==
  BHAL_outputs : Inport
  inp_CanValid_bus : Inport  Port=2
  CSCCU1 : FVT_lib/inp/can_signal_template  SystemSampleTime=-1  VariantActivationTime=update diagram  Latency=0  AutoFrameSizeCalculation=off
      link override defval: Value=KINP_CSCCU1_enum_defval
      link override ovrdflg: Value=KINP_CSCCU1_enum_ovrdflg
      link override ovrdval: Value=KINP_CSCCU1_enum_ovrdval
  DCDCAuxCur : FVT_lib/inp/can_signal_template  SystemSampleTime=-1  VariantActivationTime=update diagram  Latency=0  AutoFrameSizeCalculation=off
      link override defval: Value=KINP_DCDCAuxCur_A_defval
      link override ovrdflg: Value=KINP_DCDCAuxCur_A_ovrdflg
      link override ovrdval: Value=KINP_DCDCAuxCur_A_ovrdval
  DCDCAuxVolt : FVT_lib/inp/can_signal_template  SystemSampleTime=-1  VariantActivationTime=update diagram  Latency=0  AutoFrameSizeCalculation=off
      link override defval: Value=KINP_DCDCAuxVolt_V_defval
      link override ovrdflg: Value=KINP_DCDCAuxVolt_V_ovrdflg
      link override ovrdval: Value=KINP_DCDCAuxVolt_V_ovrdval
  DCDCHVCur : FVT_lib/inp/can_signal_template  SystemSampleTime=-1  VariantActivationTime=update diagram  Latency=0  AutoFrameSizeCalculation=off
      link override defval: Value=KINP_DCDCHVCur_A_defval
      link override ovrdflg: Value=KINP_DCDCHVCur_A_ovrdflg
      link override ovrdval: Value=KINP_DCDCHVCur_A_ovrdval
  DCDCInVoltInf : FVT_lib/inp/can_signal_template  SystemSampleTime=-1  VariantActivationTime=update diagram  Latency=0  AutoFrameSizeCalculation=off
      link override defval: Value=KINP_DCDCInVoltInf_V_defval
      link override ovrdflg: Value=KINP_DCDCInVoltInf_V_ovrdflg
      link override ovrdval: Value=KINP_DCDCInVoltInf_V_ovrdval
  DCDCPreCompleted : FVT_lib/inp/can_signal_template  SystemSampleTime=-1  VariantActivationTime=update diagram  Latency=0  AutoFrameSizeCalculation=off
      link override defval: Value=KINP_DCDCPreCompleted_enum_defval
      link override ovrdflg: Value=KINP_DCDCPreCompleted_enum_ovrdflg
      link override ovrdval: Value=KINP_DCDCPreCompleted_enum_ovrdval
  OBCDCCurrInf : FVT_lib/inp/can_signal_template  SystemSampleTime=-1  VariantActivationTime=update diagram  Latency=0  AutoFrameSizeCalculation=off
      link override defval: Value=KINP_OBCDCCurrInf_A_defval
      link override ovrdflg: Value=KINP_OBCDCCurrInf_A_ovrdflg
      link override ovrdval: Value=KINP_OBCDCCurrInf_A_ovrdval
  OBCDCVoltInf : FVT_lib/inp/can_signal_template  SystemSampleTime=-1  VariantActivationTime=update diagram  Latency=0  AutoFrameSizeCalculation=off
      link override defval: Value=KINP_OBCDCVoltInf_V_defval
      link override ovrdflg: Value=KINP_OBCDCVoltInf_V_ovrdflg
      link override ovrdval: Value=KINP_OBCDCVoltInf_V_ovrdval
  OBCPreCompleted : FVT_lib/inp/can_signal_template  SystemSampleTime=-1  VariantActivationTime=update diagram  Latency=0  AutoFrameSizeCalculation=off
      link override defval: Value=KINP_OBCPreCompleted_enum_defval
      link override ovrdflg: Value=KINP_OBCPreCompleted_enum_ovrdflg
      link override ovrdval: Value=KINP_OBCPreCompleted_enum_ovrdval
  OBCWakeup4Plugin : FVT_lib/inp/can_signal_template  SystemSampleTime=-1  VariantActivationTime=update diagram  Latency=0  AutoFrameSizeCalculation=off
      link override defval: Value=KINP_OBCWakeup4Plugin_flg_defval
      link override ovrdflg: Value=KINP_OBCWakeup4Plugin_flg_ovrdflg
      link override ovrdval: Value=KINP_OBCWakeup4Plugin_flg_ovrdval
  RCCCU1 : FVT_lib/inp/can_signal_template  SystemSampleTime=-1  VariantActivationTime=update diagram  Latency=0  AutoFrameSizeCalculation=off
      link override defval: Value=KINP_RCCCU1_enum_defval
      link override ovrdflg: Value=KINP_RCCCU1_enum_ovrdflg
      link override ovrdval: Value=KINP_RCCCU1_enum_ovrdval
  Terminator_{1..11} (11 alike) : Terminator
  True_VHAL_CSCCU1_enum : Constant  Value=TRUE  OutDataTypeStr=boolean
  True_VHAL_DCDCAuxCur_A : Constant  Value=TRUE  OutDataTypeStr=boolean
  True_VHAL_DCDCAuxVolt_V : Constant  Value=TRUE  OutDataTypeStr=boolean
  True_VHAL_DCDCHVCur_A : Constant  Value=TRUE  OutDataTypeStr=boolean
  True_VHAL_DCDCInVoltInf_V : Constant  Value=TRUE  OutDataTypeStr=boolean
  True_VHAL_DCDCPreCompleted_enum : Constant  Value=TRUE  OutDataTypeStr=boolean
  True_VHAL_OBCDCCurrInf_A : Constant  Value=TRUE  OutDataTypeStr=boolean
  True_VHAL_OBCDCVoltInf_V : Constant  Value=TRUE  OutDataTypeStr=boolean
  True_VHAL_OBCPreCompleted_enum : Constant  Value=TRUE  OutDataTypeStr=boolean
  True_VHAL_OBCWakeup4Plugin_flg : Constant  Value=TRUE  OutDataTypeStr=boolean
  True_VHAL_RCCCU1_enum : Constant  Value=TRUE  OutDataTypeStr=boolean
  slr1_{1..11} (11 alike) : BusSelector  OutputSignals=VINP_CANMsgValidCCU1_flg
  slr_VHAL_CSCCU1_enum : BusSelector  OutputSignals=VHAL_CSCCU1_enum
  slr_VHAL_DCDCAuxCur_A : BusSelector  OutputSignals=VHAL_DCDCAuxCur_A
  slr_VHAL_DCDCAuxVolt_V : BusSelector  OutputSignals=VHAL_DCDCAuxVolt_V
  slr_VHAL_DCDCHVCur_A : BusSelector  OutputSignals=VHAL_DCDCHVCur_A
  slr_VHAL_DCDCInVoltInf_V : BusSelector  OutputSignals=VHAL_DCDCInVoltInf_V
  slr_VHAL_DCDCPreCompleted_enum : BusSelector  OutputSignals=VHAL_DCDCPreCompleted_enum
  slr_VHAL_OBCDCCurrInf_A : BusSelector  OutputSignals=VHAL_OBCDCCurrInf_A
  slr_VHAL_OBCDCVoltInf_V : BusSelector  OutputSignals=VHAL_OBCDCVoltInf_V
  slr_VHAL_OBCPreCompleted_enum : BusSelector  OutputSignals=VHAL_OBCPreCompleted_enum
  slr_VHAL_OBCWakeup4Plugin_flg : BusSelector  OutputSignals=VHAL_OBCWakeup4Plugin_flg
  slr_VHAL_RCCCU1_enum : BusSelector  OutputSignals=VHAL_RCCCU1_enum
  VINP_CSCCU1_enum : Outport
  VINP_DCDCAuxCur_A : Outport  Port=2
  VINP_DCDCAuxVolt_V : Outport  Port=3
  VINP_DCDCHVCur_A : Outport  Port=4
  VINP_DCDCInVoltInf_V : Outport  Port=5
  VINP_DCDCPreCompleted_enum : Outport  Port=6
  VINP_OBCDCCurrInf_A : Outport  Port=7
  VINP_OBCDCVoltInf_V : Outport  Port=8
  VINP_OBCPreCompleted_enum : Outport  Port=9
  VINP_OBCWakeup4Plugin_flg : Outport  Port=10
  VINP_RCCCU1_enum : Outport  Port=11
  wires:
  BHAL_outputs/1 -> [BHAL_outputs]
  inp_CanValid_bus/1 -> [inp_CanValid_bus]
  [BHAL_outputs] -> slr_VHAL_CSCCU1_enum/1
  slr_VHAL_CSCCU1_enum/1 -> CSCCU1/1  "<VHAL_CSCCU1_enum>"
  True_VHAL_CSCCU1_enum/1 -> CSCCU1/2
  [inp_CanValid_bus] -> slr1_1/1
  slr1_1/1 -> CSCCU1/3  "<VINP_CANMsgValidCCU1_flg>"
  CSCCU1/1 -> VINP_CSCCU1_enum/1  "VINP_CSCCU1_enum"
  CSCCU1/2 -> Terminator_1/1
  [BHAL_outputs] -> slr_VHAL_DCDCAuxCur_A/1
  slr_VHAL_DCDCAuxCur_A/1 -> DCDCAuxCur/1  "<VHAL_DCDCAuxCur_A>"
  True_VHAL_DCDCAuxCur_A/1 -> DCDCAuxCur/2
  [inp_CanValid_bus] -> slr1_2/1
  slr1_2/1 -> DCDCAuxCur/3  "<VINP_CANMsgValidCCU1_flg>"
  DCDCAuxCur/1 -> VINP_DCDCAuxCur_A/1  "VINP_DCDCAuxCur_A"
  DCDCAuxCur/2 -> Terminator_2/1
  [BHAL_outputs] -> slr_VHAL_DCDCAuxVolt_V/1
  slr_VHAL_DCDCAuxVolt_V/1 -> DCDCAuxVolt/1  "<VHAL_DCDCAuxVolt_V>"
  True_VHAL_DCDCAuxVolt_V/1 -> DCDCAuxVolt/2
  [inp_CanValid_bus] -> slr1_3/1
  slr1_3/1 -> DCDCAuxVolt/3  "<VINP_CANMsgValidCCU1_flg>"
  DCDCAuxVolt/1 -> VINP_DCDCAuxVolt_V/1  "VINP_DCDCAuxVolt_V"
  DCDCAuxVolt/2 -> Terminator_3/1
  [BHAL_outputs] -> slr_VHAL_DCDCHVCur_A/1
  slr_VHAL_DCDCHVCur_A/1 -> DCDCHVCur/1  "<VHAL_DCDCHVCur_A>"
  True_VHAL_DCDCHVCur_A/1 -> DCDCHVCur/2
  [inp_CanValid_bus] -> slr1_4/1
  slr1_4/1 -> DCDCHVCur/3  "<VINP_CANMsgValidCCU1_flg>"
  DCDCHVCur/1 -> VINP_DCDCHVCur_A/1  "VINP_DCDCHVCur_A"
  DCDCHVCur/2 -> Terminator_4/1
  [BHAL_outputs] -> slr_VHAL_DCDCInVoltInf_V/1
  slr_VHAL_DCDCInVoltInf_V/1 -> DCDCInVoltInf/1  "<VHAL_DCDCInVoltInf_V>"
  True_VHAL_DCDCInVoltInf_V/1 -> DCDCInVoltInf/2
  [inp_CanValid_bus] -> slr1_5/1
  slr1_5/1 -> DCDCInVoltInf/3  "<VINP_CANMsgValidCCU1_flg>"
  DCDCInVoltInf/1 -> VINP_DCDCInVoltInf_V/1  "VINP_DCDCInVoltInf_V"
  DCDCInVoltInf/2 -> Terminator_5/1
  [BHAL_outputs] -> slr_VHAL_DCDCPreCompleted_enum/1
  slr_VHAL_DCDCPreCompleted_enum/1 -> DCDCPreCompleted/1  "<VHAL_DCDCPreCompleted_enum>"
  True_VHAL_DCDCPreCompleted_enum/1 -> DCDCPreCompleted/2
  [inp_CanValid_bus] -> slr1_6/1
  slr1_6/1 -> DCDCPreCompleted/3  "<VINP_CANMsgValidCCU1_flg>"
  DCDCPreCompleted/1 -> VINP_DCDCPreCompleted_enum/1  "VINP_DCDCPreCompleted_enum"
  DCDCPreCompleted/2 -> Terminator_6/1
  [BHAL_outputs] -> slr_VHAL_OBCDCCurrInf_A/1
  slr_VHAL_OBCDCCurrInf_A/1 -> OBCDCCurrInf/1  "<VHAL_OBCDCCurrInf_A>"
  True_VHAL_OBCDCCurrInf_A/1 -> OBCDCCurrInf/2
  [inp_CanValid_bus] -> slr1_7/1
  slr1_7/1 -> OBCDCCurrInf/3  "<VINP_CANMsgValidCCU1_flg>"
  OBCDCCurrInf/1 -> VINP_OBCDCCurrInf_A/1  "VINP_OBCDCCurrInf_A"
  OBCDCCurrInf/2 -> Terminator_7/1
  [BHAL_outputs] -> slr_VHAL_OBCDCVoltInf_V/1
  slr_VHAL_OBCDCVoltInf_V/1 -> OBCDCVoltInf/1  "<VHAL_OBCDCVoltInf_V>"
  True_VHAL_OBCDCVoltInf_V/1 -> OBCDCVoltInf/2
  [inp_CanValid_bus] -> slr1_8/1
  slr1_8/1 -> OBCDCVoltInf/3  "<VINP_CANMsgValidCCU1_flg>"
  OBCDCVoltInf/1 -> VINP_OBCDCVoltInf_V/1  "VINP_OBCDCVoltInf_V"
  OBCDCVoltInf/2 -> Terminator_8/1
  [BHAL_outputs] -> slr_VHAL_OBCPreCompleted_enum/1
  slr_VHAL_OBCPreCompleted_enum/1 -> OBCPreCompleted/1  "<VHAL_OBCPreCompleted_enum>"
  True_VHAL_OBCPreCompleted_enum/1 -> OBCPreCompleted/2
  [inp_CanValid_bus] -> slr1_9/1
  slr1_9/1 -> OBCPreCompleted/3  "<VINP_CANMsgValidCCU1_flg>"
  OBCPreCompleted/1 -> VINP_OBCPreCompleted_enum/1  "VINP_OBCPreCompleted_enum"
  OBCPreCompleted/2 -> Terminator_9/1
  [BHAL_outputs] -> slr_VHAL_OBCWakeup4Plugin_flg/1
  slr_VHAL_OBCWakeup4Plugin_flg/1 -> OBCWakeup4Plugin/1  "<VHAL_OBCWakeup4Plugin_flg>"
  True_VHAL_OBCWakeup4Plugin_flg/1 -> OBCWakeup4Plugin/2
  [inp_CanValid_bus] -> slr1_10/1
  slr1_10/1 -> OBCWakeup4Plugin/3  "<VINP_CANMsgValidCCU1_flg>"
  OBCWakeup4Plugin/1 -> VINP_OBCWakeup4Plugin_flg/1  "VINP_OBCWakeup4Plugin_flg"
  OBCWakeup4Plugin/2 -> Terminator_10/1
  [BHAL_outputs] -> slr_VHAL_RCCCU1_enum/1
  slr_VHAL_RCCCU1_enum/1 -> RCCCU1/1  "<VHAL_RCCCU1_enum>"
  True_VHAL_RCCCU1_enum/1 -> RCCCU1/2
  [inp_CanValid_bus] -> slr1_11/1
  slr1_11/1 -> RCCCU1/3  "<VINP_CANMsgValidCCU1_flg>"
  RCCCU1/1 -> VINP_RCCCU1_enum/1  "VINP_RCCCU1_enum"
  RCCCU1/2 -> Terminator_11/1

== system inp/INP/CAN3/SignalCheck/CCU2 ==
  BHAL_outputs : Inport
  inp_CanValid_bus : Inport  Port=2
  CSCCU2 : FVT_lib/inp/can_signal_template  SystemSampleTime=-1  VariantActivationTime=update diagram  Latency=0  AutoFrameSizeCalculation=off
      link override defval: Value=KINP_CSCCU2_enum_defval
      link override ovrdflg: Value=KINP_CSCCU2_enum_ovrdflg
      link override ovrdval: Value=KINP_CSCCU2_enum_ovrdval
  DCDCEnaSta : FVT_lib/inp/can_signal_template  SystemSampleTime=-1  VariantActivationTime=update diagram  Latency=0  AutoFrameSizeCalculation=off
      link override defval: Value=KINP_DCDCEnaSta_flg_defval
      link override ovrdflg: Value=KINP_DCDCEnaSta_flg_ovrdflg
      link override ovrdval: Value=KINP_DCDCEnaSta_flg_ovrdval
  DCDCFaultSta : FVT_lib/inp/can_signal_template  SystemSampleTime=-1  VariantActivationTime=update diagram  Latency=0  AutoFrameSizeCalculation=off
      link override defval: Value=KINP_DCDCFaultSta_enum_defval
      link override ovrdflg: Value=KINP_DCDCFaultSta_enum_ovrdflg
      link override ovrdval: Value=KINP_DCDCFaultSta_enum_ovrdval
  DCDCReady4Pre : FVT_lib/inp/can_signal_template  SystemSampleTime=-1  VariantActivationTime=update diagram  Latency=0  AutoFrameSizeCalculation=off
      link override defval: Value=KINP_DCDCReady4Pre_flg_defval
      link override ovrdflg: Value=KINP_DCDCReady4Pre_flg_ovrdflg
      link override ovrdval: Value=KINP_DCDCReady4Pre_flg_ovrdval
  DCDCTemp : FVT_lib/inp/can_signal_template  SystemSampleTime=-1  VariantActivationTime=update diagram  Latency=0  AutoFrameSizeCalculation=off
      link override defval: Value=KINP_DCDCTemp_C_defval
      link override ovrdflg: Value=KINP_DCDCTemp_C_ovrdflg
      link override ovrdval: Value=KINP_DCDCTemp_C_ovrdval
  OBCACCurLim : FVT_lib/inp/can_signal_template  SystemSampleTime=-1  VariantActivationTime=update diagram  Latency=0  AutoFrameSizeCalculation=off
      link override defval: Value=KINP_OBCACCurLim_enum_defval
      link override ovrdflg: Value=KINP_OBCACCurLim_enum_ovrdflg
      link override ovrdval: Value=KINP_OBCACCurLim_enum_ovrdval
  OBCACCurrInf : FVT_lib/inp/can_signal_template  SystemSampleTime=-1  VariantActivationTime=update diagram  Latency=0  AutoFrameSizeCalculation=off
      link override defval: Value=KINP_OBCACCurrInf_A_defval
      link override ovrdflg: Value=KINP_OBCACCurrInf_A_ovrdflg
      link override ovrdval: Value=KINP_OBCACCurrInf_A_ovrdval
  OBCACVoltInf : FVT_lib/inp/can_signal_template  SystemSampleTime=-1  VariantActivationTime=update diagram  Latency=0  AutoFrameSizeCalculation=off
      link override defval: Value=KINP_OBCACVoltInf_V_defval
      link override ovrdflg: Value=KINP_OBCACVoltInf_V_ovrdflg
      link override ovrdval: Value=KINP_OBCACVoltInf_V_ovrdval
  OBCEnaSta : FVT_lib/inp/can_signal_template  SystemSampleTime=-1  VariantActivationTime=update diagram  Latency=0  AutoFrameSizeCalculation=off
      link override defval: Value=KINP_OBCEnaSta_flg_defval
      link override ovrdflg: Value=KINP_OBCEnaSta_flg_ovrdflg
      link override ovrdval: Value=KINP_OBCEnaSta_flg_ovrdval
  OBCFaultSta : FVT_lib/inp/can_signal_template  SystemSampleTime=-1  VariantActivationTime=update diagram  Latency=0  AutoFrameSizeCalculation=off
      link override defval: Value=KINP_OBCFaultSta_enum_defval
      link override ovrdflg: Value=KINP_OBCFaultSta_enum_ovrdflg
      link override ovrdval: Value=KINP_OBCFaultSta_enum_ovrdval
  OBCPluginSta : FVT_lib/inp/can_signal_template  SystemSampleTime=-1  VariantActivationTime=update diagram  Latency=0  AutoFrameSizeCalculation=off
      link override defval: Value=KINP_OBCPluginSta_flg_defval
      link override ovrdflg: Value=KINP_OBCPluginSta_flg_ovrdflg
      link override ovrdval: Value=KINP_OBCPluginSta_flg_ovrdval
  OBCReady4Pre : FVT_lib/inp/can_signal_template  SystemSampleTime=-1  VariantActivationTime=update diagram  Latency=0  AutoFrameSizeCalculation=off
      link override defval: Value=KINP_OBCReady4Pre_flg_defval
      link override ovrdflg: Value=KINP_OBCReady4Pre_flg_ovrdflg
      link override ovrdval: Value=KINP_OBCReady4Pre_flg_ovrdval
  OBCTemp : FVT_lib/inp/can_signal_template  SystemSampleTime=-1  VariantActivationTime=update diagram  Latency=0  AutoFrameSizeCalculation=off
      link override defval: Value=KINP_OBCTemp_C_defval
      link override ovrdflg: Value=KINP_OBCTemp_C_ovrdflg
      link override ovrdval: Value=KINP_OBCTemp_C_ovrdval
  OBCV2LSta : FVT_lib/inp/can_signal_template  SystemSampleTime=-1  VariantActivationTime=update diagram  Latency=0  AutoFrameSizeCalculation=off
      link override defval: Value=KINP_OBCV2LSta_enum_defval
      link override ovrdflg: Value=KINP_OBCV2LSta_enum_ovrdflg
      link override ovrdval: Value=KINP_OBCV2LSta_enum_ovrdval
  RCCCU2 : FVT_lib/inp/can_signal_template  SystemSampleTime=-1  VariantActivationTime=update diagram  Latency=0  AutoFrameSizeCalculation=off
      link override defval: Value=KINP_RCCCU2_enum_defval
      link override ovrdflg: Value=KINP_RCCCU2_enum_ovrdflg
      link override ovrdval: Value=KINP_RCCCU2_enum_ovrdval
  Terminator_{1..15} (15 alike) : Terminator
  True_VHAL_CSCCU2_enum : Constant  Value=TRUE  OutDataTypeStr=boolean
  True_VHAL_DCDCEnaSta_flg : Constant  Value=TRUE  OutDataTypeStr=boolean
  True_VHAL_DCDCFaultSta_enum : Constant  Value=TRUE  OutDataTypeStr=boolean
  True_VHAL_DCDCReady4Pre_flg : Constant  Value=TRUE  OutDataTypeStr=boolean
  True_VHAL_DCDCTemp_C : Constant  Value=TRUE  OutDataTypeStr=boolean
  True_VHAL_OBCACCurLim_enum : Constant  Value=TRUE  OutDataTypeStr=boolean
  True_VHAL_OBCACCurrInf_A : Constant  Value=TRUE  OutDataTypeStr=boolean
  True_VHAL_OBCACVoltInf_V : Constant  Value=TRUE  OutDataTypeStr=boolean
  True_VHAL_OBCEnaSta_flg : Constant  Value=TRUE  OutDataTypeStr=boolean
  True_VHAL_OBCFaultSta_enum : Constant  Value=TRUE  OutDataTypeStr=boolean
  True_VHAL_OBCPluginSta_flg : Constant  Value=TRUE  OutDataTypeStr=boolean
  True_VHAL_OBCReady4Pre_flg : Constant  Value=TRUE  OutDataTypeStr=boolean
  True_VHAL_OBCTemp_C : Constant  Value=TRUE  OutDataTypeStr=boolean
  True_VHAL_OBCV2LSta_enum : Constant  Value=TRUE  OutDataTypeStr=boolean
  True_VHAL_RCCCU2_enum : Constant  Value=TRUE  OutDataTypeStr=boolean
  slr1_{1..15} (15 alike) : BusSelector  OutputSignals=VINP_CANMsgValidCCU2_flg
  slr_VHAL_CSCCU2_enum : BusSelector  OutputSignals=VHAL_CSCCU2_enum
  slr_VHAL_DCDCEnaSta_flg : BusSelector  OutputSignals=VHAL_DCDCEnaSta_flg
  slr_VHAL_DCDCFaultSta_enum : BusSelector  OutputSignals=VHAL_DCDCFaultSta_enum
  slr_VHAL_DCDCReady4Pre_flg : BusSelector  OutputSignals=VHAL_DCDCReady4Pre_flg
  slr_VHAL_DCDCTemp_C : BusSelector  OutputSignals=VHAL_DCDCTemp_C
  slr_VHAL_OBCACCurLim_enum : BusSelector  OutputSignals=VHAL_OBCACCurLim_enum
  slr_VHAL_OBCACCurrInf_A : BusSelector  OutputSignals=VHAL_OBCACCurrInf_A
  slr_VHAL_OBCACVoltInf_V : BusSelector  OutputSignals=VHAL_OBCACVoltInf_V
  slr_VHAL_OBCEnaSta_flg : BusSelector  OutputSignals=VHAL_OBCEnaSta_flg
  slr_VHAL_OBCFaultSta_enum : BusSelector  OutputSignals=VHAL_OBCFaultSta_enum
  slr_VHAL_OBCPluginSta_flg : BusSelector  OutputSignals=VHAL_OBCPluginSta_flg
  slr_VHAL_OBCReady4Pre_flg : BusSelector  OutputSignals=VHAL_OBCReady4Pre_flg
  slr_VHAL_OBCTemp_C : BusSelector  OutputSignals=VHAL_OBCTemp_C
  slr_VHAL_OBCV2LSta_enum : BusSelector  OutputSignals=VHAL_OBCV2LSta_enum
  slr_VHAL_RCCCU2_enum : BusSelector  OutputSignals=VHAL_RCCCU2_enum
  VINP_CSCCU2_enum : Outport
  VINP_DCDCEnaSta_flg : Outport  Port=2
  VINP_DCDCFaultSta_enum : Outport  Port=3
  VINP_DCDCReady4Pre_flg : Outport  Port=4
  VINP_DCDCTemp_C : Outport  Port=5
  VINP_OBCACCurrInf_A : Outport  Port=6
  VINP_OBCACVoltInf_V : Outport  Port=7
  VINP_OBCEnaSta_flg : Outport  Port=8
  VINP_OBCFaultSta_enum : Outport  Port=9
  VINP_OBCPluginSta_flg : Outport  Port=10
  VINP_OBCReady4Pre_flg : Outport  Port=11
  VINP_OBCTemp_C : Outport  Port=12
  VINP_OBCV2LSta_enum : Outport  Port=13
  VINP_OBCACCurLim_enum : Outport  Port=14
  VINP_RCCCU2_enum : Outport  Port=15
  wires:
  BHAL_outputs/1 -> [BHAL_outputs]
  inp_CanValid_bus/1 -> [inp_CanValid_bus]
  [BHAL_outputs] -> slr_VHAL_CSCCU2_enum/1
  slr_VHAL_CSCCU2_enum/1 -> CSCCU2/1  "<VHAL_CSCCU2_enum>"
  True_VHAL_CSCCU2_enum/1 -> CSCCU2/2
  [inp_CanValid_bus] -> slr1_1/1
  slr1_1/1 -> CSCCU2/3  "<VINP_CANMsgValidCCU2_flg>"
  CSCCU2/1 -> VINP_CSCCU2_enum/1  "VINP_CSCCU2_enum"
  CSCCU2/2 -> Terminator_1/1
  [BHAL_outputs] -> slr_VHAL_DCDCEnaSta_flg/1
  slr_VHAL_DCDCEnaSta_flg/1 -> DCDCEnaSta/1  "<VHAL_DCDCEnaSta_flg>"
  True_VHAL_DCDCEnaSta_flg/1 -> DCDCEnaSta/2
  [inp_CanValid_bus] -> slr1_2/1
  slr1_2/1 -> DCDCEnaSta/3  "<VINP_CANMsgValidCCU2_flg>"
  DCDCEnaSta/1 -> VINP_DCDCEnaSta_flg/1  "VINP_DCDCEnaSta_flg"
  DCDCEnaSta/2 -> Terminator_2/1
  [BHAL_outputs] -> slr_VHAL_DCDCFaultSta_enum/1
  slr_VHAL_DCDCFaultSta_enum/1 -> DCDCFaultSta/1  "<VHAL_DCDCFaultSta_enum>"
  True_VHAL_DCDCFaultSta_enum/1 -> DCDCFaultSta/2
  [inp_CanValid_bus] -> slr1_3/1
  slr1_3/1 -> DCDCFaultSta/3  "<VINP_CANMsgValidCCU2_flg>"
  DCDCFaultSta/1 -> VINP_DCDCFaultSta_enum/1  "VINP_DCDCFaultSta_enum"
  DCDCFaultSta/2 -> Terminator_3/1
  [BHAL_outputs] -> slr_VHAL_DCDCReady4Pre_flg/1
  slr_VHAL_DCDCReady4Pre_flg/1 -> DCDCReady4Pre/1  "<VHAL_DCDCReady4Pre_flg>"
  True_VHAL_DCDCReady4Pre_flg/1 -> DCDCReady4Pre/2
  [inp_CanValid_bus] -> slr1_4/1
  slr1_4/1 -> DCDCReady4Pre/3  "<VINP_CANMsgValidCCU2_flg>"
  DCDCReady4Pre/1 -> VINP_DCDCReady4Pre_flg/1  "VINP_DCDCReady4Pre_flg"
  DCDCReady4Pre/2 -> Terminator_4/1
  [BHAL_outputs] -> slr_VHAL_DCDCTemp_C/1
  slr_VHAL_DCDCTemp_C/1 -> DCDCTemp/1  "<VHAL_DCDCTemp_C>"
  True_VHAL_DCDCTemp_C/1 -> DCDCTemp/2
  [inp_CanValid_bus] -> slr1_5/1
  slr1_5/1 -> DCDCTemp/3  "<VINP_CANMsgValidCCU2_flg>"
  DCDCTemp/1 -> VINP_DCDCTemp_C/1  "VINP_DCDCTemp_C"
  DCDCTemp/2 -> Terminator_5/1
  [BHAL_outputs] -> slr_VHAL_OBCACCurrInf_A/1
  slr_VHAL_OBCACCurrInf_A/1 -> OBCACCurrInf/1  "<VHAL_OBCACCurrInf_A>"
  True_VHAL_OBCACCurrInf_A/1 -> OBCACCurrInf/2
  [inp_CanValid_bus] -> slr1_6/1
  slr1_6/1 -> OBCACCurrInf/3  "<VINP_CANMsgValidCCU2_flg>"
  OBCACCurrInf/1 -> VINP_OBCACCurrInf_A/1  "VINP_OBCACCurrInf_A"
  OBCACCurrInf/2 -> Terminator_6/1
  [BHAL_outputs] -> slr_VHAL_OBCACVoltInf_V/1
  slr_VHAL_OBCACVoltInf_V/1 -> OBCACVoltInf/1  "<VHAL_OBCACVoltInf_V>"
  True_VHAL_OBCACVoltInf_V/1 -> OBCACVoltInf/2
  [inp_CanValid_bus] -> slr1_7/1
  slr1_7/1 -> OBCACVoltInf/3  "<VINP_CANMsgValidCCU2_flg>"
  OBCACVoltInf/1 -> VINP_OBCACVoltInf_V/1  "VINP_OBCACVoltInf_V"
  OBCACVoltInf/2 -> Terminator_7/1
  [BHAL_outputs] -> slr_VHAL_OBCEnaSta_flg/1
  slr_VHAL_OBCEnaSta_flg/1 -> OBCEnaSta/1  "<VHAL_OBCEnaSta_flg>"
  True_VHAL_OBCEnaSta_flg/1 -> OBCEnaSta/2
  [inp_CanValid_bus] -> slr1_8/1
  slr1_8/1 -> OBCEnaSta/3  "<VINP_CANMsgValidCCU2_flg>"
  OBCEnaSta/1 -> VINP_OBCEnaSta_flg/1  "VINP_OBCEnaSta_flg"
  OBCEnaSta/2 -> Terminator_8/1
  [BHAL_outputs] -> slr_VHAL_OBCFaultSta_enum/1
  slr_VHAL_OBCFaultSta_enum/1 -> OBCFaultSta/1  "<VHAL_OBCFaultSta_enum>"
  True_VHAL_OBCFaultSta_enum/1 -> OBCFaultSta/2
  [inp_CanValid_bus] -> slr1_9/1
  slr1_9/1 -> OBCFaultSta/3  "<VINP_CANMsgValidCCU2_flg>"
  OBCFaultSta/1 -> VINP_OBCFaultSta_enum/1  "VINP_OBCFaultSta_enum"
  OBCFaultSta/2 -> Terminator_9/1
  [BHAL_outputs] -> slr_VHAL_OBCPluginSta_flg/1
  slr_VHAL_OBCPluginSta_flg/1 -> OBCPluginSta/1  "<VHAL_OBCPluginSta_flg>"
  True_VHAL_OBCPluginSta_flg/1 -> OBCPluginSta/2
  [inp_CanValid_bus] -> slr1_10/1
  slr1_10/1 -> OBCPluginSta/3  "<VINP_CANMsgValidCCU2_flg>"
  OBCPluginSta/1 -> VINP_OBCPluginSta_flg/1  "VINP_OBCPluginSta_flg"
  OBCPluginSta/2 -> Terminator_10/1
  [BHAL_outputs] -> slr_VHAL_OBCReady4Pre_flg/1
  slr_VHAL_OBCReady4Pre_flg/1 -> OBCReady4Pre/1  "<VHAL_OBCReady4Pre_flg>"
  True_VHAL_OBCReady4Pre_flg/1 -> OBCReady4Pre/2
  [inp_CanValid_bus] -> slr1_11/1
  slr1_11/1 -> OBCReady4Pre/3  "<VINP_CANMsgValidCCU2_flg>"
  OBCReady4Pre/1 -> VINP_OBCReady4Pre_flg/1  "VINP_OBCReady4Pre_flg"
  OBCReady4Pre/2 -> Terminator_11/1
  [BHAL_outputs] -> slr_VHAL_OBCTemp_C/1
  slr_VHAL_OBCTemp_C/1 -> OBCTemp/1  "<VHAL_OBCTemp_C>"
  True_VHAL_OBCTemp_C/1 -> OBCTemp/2
  [inp_CanValid_bus] -> slr1_12/1
  slr1_12/1 -> OBCTemp/3  "<VINP_CANMsgValidCCU2_flg>"
  OBCTemp/1 -> VINP_OBCTemp_C/1  "VINP_OBCTemp_C"
  OBCTemp/2 -> Terminator_12/1
  [BHAL_outputs] -> slr_VHAL_OBCV2LSta_enum/1
  slr_VHAL_OBCV2LSta_enum/1 -> OBCV2LSta/1  "<VHAL_OBCV2LSta_enum>"
  True_VHAL_OBCV2LSta_enum/1 -> OBCV2LSta/2
  [inp_CanValid_bus] -> slr1_13/1
  slr1_13/1 -> OBCV2LSta/3  "<VINP_CANMsgValidCCU2_flg>"
  OBCV2LSta/1 -> VINP_OBCV2LSta_enum/1  "VINP_OBCV2LSta_enum"
  OBCV2LSta/2 -> Terminator_13/1
  [BHAL_outputs] -> slr_VHAL_OBCACCurLim_enum/1
  slr_VHAL_OBCACCurLim_enum/1 -> OBCACCurLim/1  "<VHAL_OBCACCurLim_enum>"
  True_VHAL_OBCACCurLim_enum/1 -> OBCACCurLim/2
  [inp_CanValid_bus] -> slr1_14/1
  slr1_14/1 -> OBCACCurLim/3  "<VINP_CANMsgValidCCU2_flg>"
  OBCACCurLim/1 -> VINP_OBCACCurLim_enum/1  "VINP_OBCACCurLim_enum"
  OBCACCurLim/2 -> Terminator_14/1
  [BHAL_outputs] -> slr_VHAL_RCCCU2_enum/1
  slr_VHAL_RCCCU2_enum/1 -> RCCCU2/1  "<VHAL_RCCCU2_enum>"
  True_VHAL_RCCCU2_enum/1 -> RCCCU2/2
  [inp_CanValid_bus] -> slr1_15/1
  slr1_15/1 -> RCCCU2/3  "<VINP_CANMsgValidCCU2_flg>"
  RCCCU2/1 -> VINP_RCCCU2_enum/1  "VINP_RCCCU2_enum"
  RCCCU2/2 -> Terminator_15/1
